simulink model "sTargetFinder"  (R2022a)
settings: Solver=VariableStepAuto  StartTime=0.0  StopTime=1.0  RelTol=1e-3
undefined symbols (not defined in the file): conv_len, photoA, photoB, thres
libraries: visionanalysis x2, visionfilter x1, dspstat3 x1
settings Model: Creator=iacca  LastModifiedBy=iacca

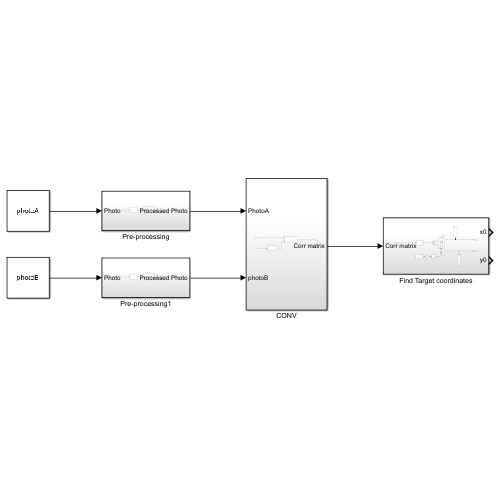
[thumbnail: Simulink's stored preview of the top-level diagram]
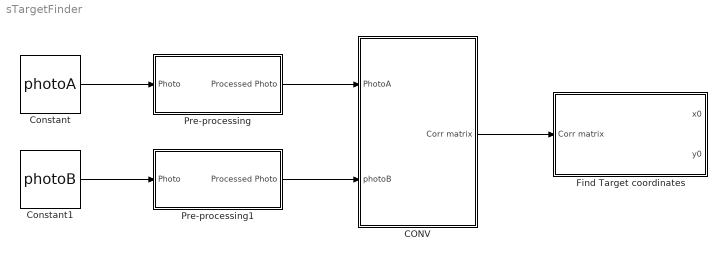
== system sTargetFinder ==
  CONV : Subsystem
  Constant : Constant  Value=photoA  VectorParams1D=off
  Constant1 : Constant  Value=photoB  VectorParams1D=off
  Find Target coordinates : Subsystem
  Pre-processing : Subsystem
  Pre-processing1 : Subsystem
  wires:
  Constant/1 -> Pre-processing/1(Photo)
  Constant1/1 -> Pre-processing1/1(Photo)
  Pre-processing/1(Processed Photo) -> CONV/1(PhotoA)
  Pre-processing1/1(Processed Photo) -> CONV/2(photoB)
  CONV/1(Corr matrix) -> Find Target coordinates/1(Corr matrix)

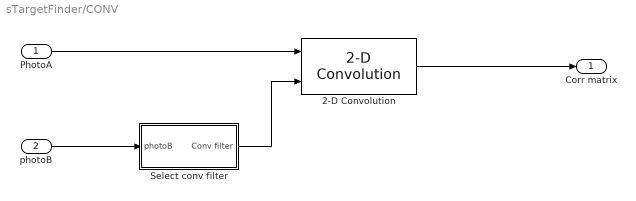
== system sTargetFinder/CONV ==
  PhotoA : Inport
  photoB : Inport  Port=2
  2-D Convolution : visionfilter/2-D Convolution  outSize=Same as input port I1  normalize=off  roundingMode=Nearest  overflowMode=off
      settings: SourceProductBaseCode=VP
  Select conv filter : Subsystem
  Corr matrix : Outport
  wires:
  Select conv filter/1(Conv filter) -> 2-D Convolution/2
  PhotoA/1 -> 2-D Convolution/1
  photoB/1 -> Select conv filter/1(photoB)
  2-D Convolution/1 -> Corr matrix/1

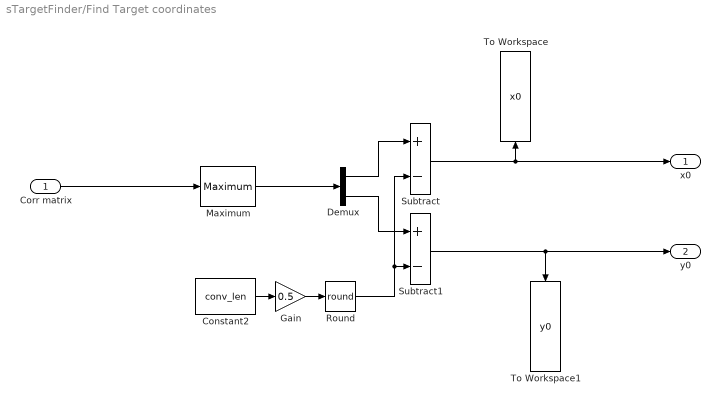
== system sTargetFinder/Find Target coordinates ==
  Corr matrix : Inport
  Constant2 : Constant  Value=conv_len
  Demux : Demux  Outputs=2
  Gain : Gain  Gain=0.5
  Maximum : dspstat3/Maximum  operation=maximum  fcn=Index  indexBase=One  operateOver=Entire input  Dimension=1  InputProcessing=Columns as channels (frame based)  reset=None  roiEnable=off  roiType=Rectangles  roiPortion=Entire ROI  roiOutput=Individual statistics for each ROI  roiFlag=off  roundingMode=Floor  overflowMode=off  accumDataTypeStr=Inherit: Same as product output  accumLastDataTypeStr=Inherit: Same as product output
  Round : Rounding  Operator=round
  Subtract : Sum  Inputs=+-
  Subtract1 : Sum  Inputs=+-
  To Workspace : ToWorkspace  VariableName=x0  SampleTime=-1
  To Workspace1 : ToWorkspace  VariableName=y0  SampleTime=-1
  x0 : Outport
  y0 : Outport  Port=2
  wires:
  Demux/2 -> Subtract1/1
  Maximum/1 -> Demux/1
  Round/1 -> Subtract1/2, Subtract/2
  Corr matrix/1 -> Maximum/1
  Subtract/1 -> x0/1, To Workspace/1
  Gain/1 -> Round/1
  Constant2/1 -> Gain/1
  Demux/1 -> Subtract/1
  Subtract1/1 -> y0/1, To Workspace1/1

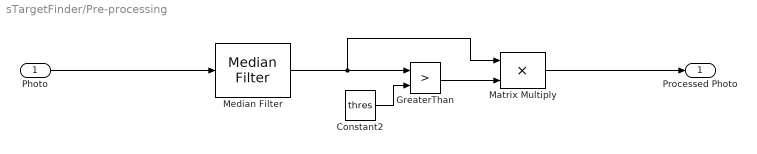
== system sTargetFinder/Pre-processing ==
  Photo : Inport
  Constant2 : Constant  Value=thres
  GreaterThan : RelationalOperator  Operator=>  OutDataTypeStr=boolean  RndMeth=Simplest  InputSameDT=off
  Matrix Multiply : Product
  Median Filter : visionanalysis/Median Filter  nghbood=[3 3]  outSize=Same as input port I  padType=Symmetric  padSrc=Specify via dialog  padVal=0  roundingMode=Floor  overflowMode=off
      settings: SourceProductBaseCode=VP
  Processed Photo : Outport
  wires:
  Median Filter/1 -> Matrix Multiply/1, GreaterThan/1
  Constant2/1 -> GreaterThan/2
  GreaterThan/1 -> Matrix Multiply/2
  Matrix Multiply/1 -> Processed Photo/1
  Photo/1 -> Median Filter/1

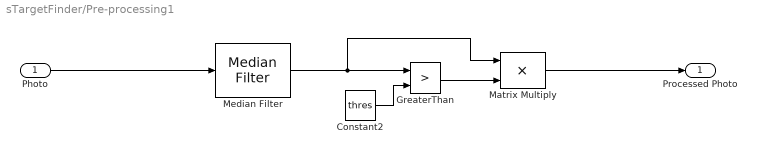
== system sTargetFinder/Pre-processing1 ==
  Photo : Inport
  Constant2 : Constant  Value=thres
  GreaterThan : RelationalOperator  Operator=>  OutDataTypeStr=boolean  RndMeth=Simplest  InputSameDT=off
  Matrix Multiply : Product
  Median Filter : visionanalysis/Median Filter  nghbood=[3 3]  outSize=Same as input port I  padType=Symmetric  padSrc=Specify via dialog  padVal=0  roundingMode=Floor  overflowMode=off
      settings: SourceProductBaseCode=VP
  Processed Photo : Outport
  wires:
  Median Filter/1 -> Matrix Multiply/1, GreaterThan/1
  Constant2/1 -> GreaterThan/2
  GreaterThan/1 -> Matrix Multiply/2
  Matrix Multiply/1 -> Processed Photo/1
  Photo/1 -> Median Filter/1

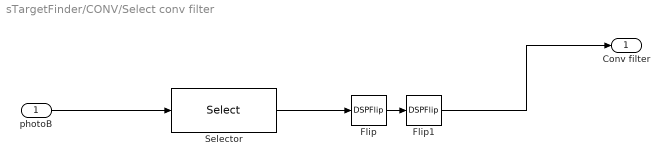
== system sTargetFinder/CONV/Select conv filter ==
  photoB : Inport
  Flip : DSPFlip
  Flip1 : DSPFlip  dim=Rows
  Selector : Selector  NumberOfDimensions=2  InputPortWidth=3  IndexOptions=Index vector (dialog),Index vector (dialog)  Indices=[1:conv_len],[1:conv_len]  OutputSizes=1,1
  Conv filter : Outport
  wires:
  Flip/1 -> Flip1/1
  Selector/1 -> Flip/1
  photoB/1 -> Selector/1
  Flip1/1 -> Conv filter/1
